simulink model "Test_model_nou"  (R2023b)
settings: Solver=ode15s  StartTime=0.0  StopTime=10  RelTol=1e-3
values from neighbouring files (symbols this model uses):
  Ts = 0.1    [NonLinearARXModel.mat]    (also in NonLinearHammerstein-Weiner.mat; Workspace.mat)
settings Model: Creator=petri  LastModifiedBy=petri

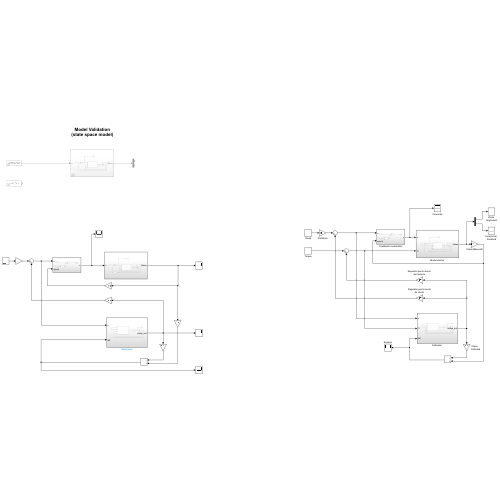
[thumbnail: Simulink's stored preview of the top-level diagram]
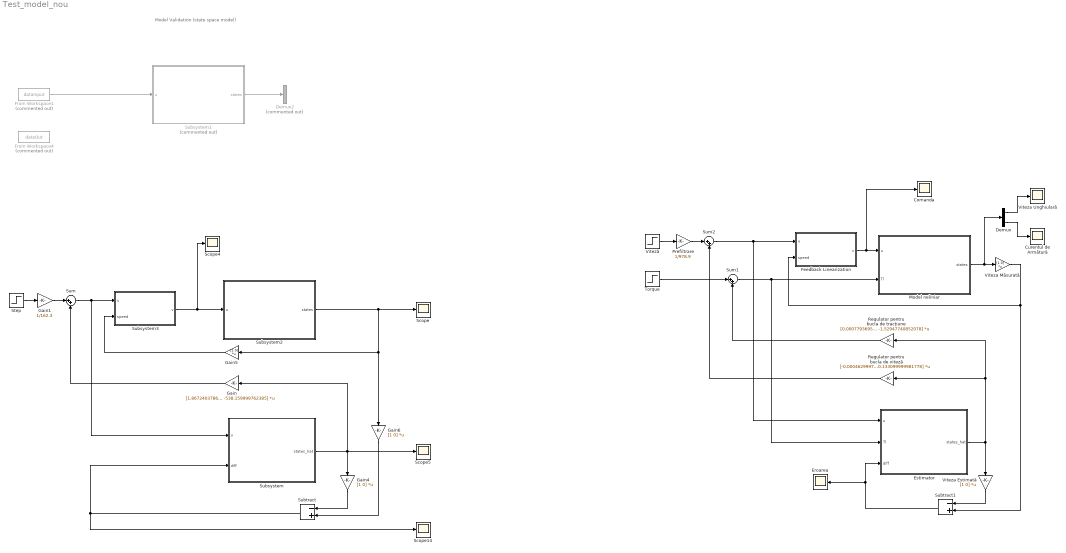
== system Test_model_nou ==
  note: Model Validation
      | (state space model)
  Comanda : Scope
  Curentul de Armătură : Scope
  Demux : Demux  Outputs=2
  Demux2 : Demux  Commented=on  Outputs=2
  Eroarea : Scope
  "Estimator " : Subsystem
  Feedback Linearization : Subsystem
  From Workspace1 : FromWorkspace  Commented=on  VariableName=dataInput  SampleTime=Ts
  From Workspace4 : FromWorkspace  Commented=on  VariableName=dataOut  SampleTime=Ts
  Gain : Gain  Gain=[1.86724037861208 -538.159999762385]  Multiplication=Matrix(K*u)
  Gain1 : Gain  Gain=1/162.3
  Gain4 : Gain  Gain=[1 0]  Multiplication=Matrix(K*u)
  Gain5 : Gain  Gain=[1 0]  Multiplication=Matrix(K*u)
  Gain6 : Gain  Gain=[1 0]  Multiplication=Matrix(K*u)
  Model neliniar : Subsystem
  Prefiltrare : Gain  Gain=1/978.9
  Regulator pentru bucla de viteză : Gain  Gain="[-0.000462999781953050\t0.133099999981778]"  Multiplication=Matrix(K*u)
  Regulator pentru bucla de tracțiune : Gain  Gain="[0.000779369551615828\t-1.52947740852078]"  Multiplication=Matrix(K*u)
  Scope{,4..5,14} (4 alike) : Scope
  Step : Step  Time=0  After=200  SampleTime=0
  Subsystem : Subsystem
  Subsystem1 : Subsystem  Commented=on
  Subsystem2 : Subsystem
  Subsystem3 : Subsystem
  Subtract : Sum  Inputs=-+
  Subtract1 : Sum  Inputs=-+
  Sum : Sum  Inputs=|++
  Sum1 : Sum  Inputs=|++
  Sum2 : Sum  Inputs=|++
  Torque : Step  Time=5  After=0.05  SampleTime=0
  Viteza Estimată : Gain  Gain=[1 0]  Multiplication=Matrix(K*u)
  Viteza Unghiulară : Scope
  Viteza Măsurată : Gain  Gain=[1 0]  Multiplication=Matrix(K*u)
  Viteză : Step  Time=0  After=160  SampleTime=0
  wires:
  From Workspace1/1 -> Subsystem1/1(u)
  Subsystem1/1(states) -> Demux2/1
  Subsystem3/1(v) -> Scope4/1, Subsystem2/1(u)
  Subsystem2/1(states) -> Scope/1, Gain6/1, Gain5/1
  Sum/1 -> Subsystem3/1(u), Subsystem/1(u)
  Gain/1 -> Sum/2
  Gain5/1 -> Subsystem3/2(speed)
  Subsystem/1(states_hat) -> Gain/1, Scope5/1, Gain4/1
  Gain4/1 -> Subtract/1
  Gain6/1 -> Subtract/2
  Subtract/1 -> Subsystem/2(diff), Scope14/1
  Step/1 -> Gain1/1
  Gain1/1 -> Sum/1
  Feedback Linearization/1(v) -> Model neliniar/1(u), Comanda/1
  Model neliniar/1(states) -> Viteza Măsurată/1, Demux/1
  Sum1/1 -> Model neliniar/2(Tl), "Estimator "/2(Tl)
  Sum2/1 -> "Estimator "/1(u), Feedback Linearization/1(u)
  Regulator pentru bucla de viteză/1 -> Sum2/2
  "Estimator "/1(states_hat) -> Viteza Estimată/1, Regulator pentru bucla de viteză/1, Regulator pentru bucla de tracțiune/1
  Viteza Estimată/1 -> Subtract1/1
  Viteza Măsurată/1 -> Feedback Linearization/2(speed), Subtract1/2
  Subtract1/1 -> Eroarea/1, "Estimator "/3(diff)
  Viteză/1 -> Prefiltrare/1
  Prefiltrare/1 -> Sum2/1
  Demux/1 -> Viteza Unghiulară/1
  Demux/2 -> Curentul de Armătură/1
  Regulator pentru bucla de tracțiune/1 -> Sum1/2
  Torque/1 -> Sum1/1

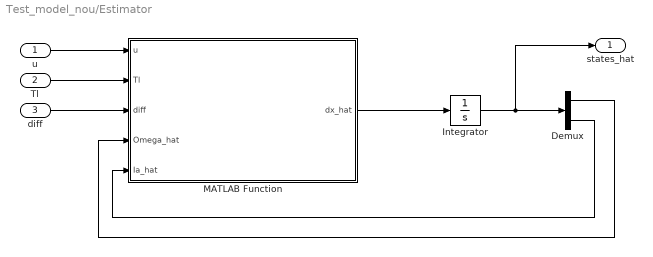
== system Test_model_nou/Estimator  ==
  u : Inport
  Tl : Inport  Port=2
  diff : Inport  Port=3
  Demux : Demux  Outputs=2
  Integrator : Integrator
  MATLAB Function : MATLAB Function  TreatAsAtomicUnit=on
  states_hat : Outport
  wires:
  u/1 -> MATLAB Function/1(u)
  Integrator/1 -> states_hat/1, Demux/1
  MATLAB Function/1(dx_hat) -> Integrator/1
  diff/1 -> MATLAB Function/3(diff)
  Demux/1 -> MATLAB Function/4(Omega_hat)
  Demux/2 -> MATLAB Function/5(Ia_hat)
  Tl/1 -> MATLAB Function/2(Tl)

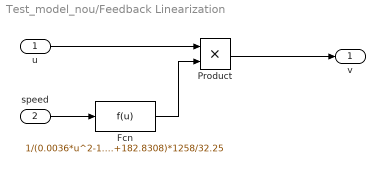
== system Test_model_nou/Feedback Linearization ==
  u : Inport
  speed : Inport  Port=2
  Fcn : Fcn  Expr=1/(0.0036*u^2-1.4479*u+182.8308)*1258/32.25
  Product : Product
  v : Outport
  wires:
  u/1 -> Product/1
  Fcn/1 -> Product/2
  speed/1 -> Fcn/1
  Product/1 -> v/1

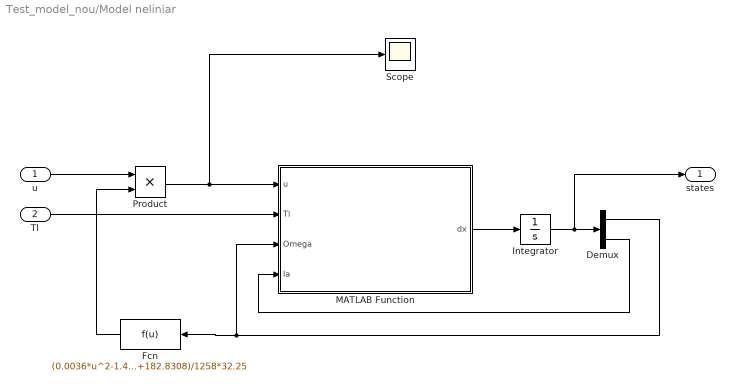
== system Test_model_nou/Model neliniar ==
  u : Inport
  Tl : Inport  Port=2
  Demux : Demux  Outputs=2
  Fcn : Fcn  Expr=(0.0036*u^2-1.4479*u+182.8308)/1258*32.25
  Integrator : Integrator
  MATLAB Function : MATLAB Function  TreatAsAtomicUnit=on
  Product : Product
  Scope : Scope
  states : Outport
  wires:
  Integrator/1 -> states/1, Demux/1
  Demux/2 -> MATLAB Function/4(Ia)
  MATLAB Function/1(dx) -> Integrator/1
  Demux/1 -> Fcn/1, MATLAB Function/3(Omega)
  u/1 -> Product/1
  Product/1 -> Scope/1, MATLAB Function/1(u)
  Fcn/1 -> Product/2
  Tl/1 -> MATLAB Function/2(Tl)

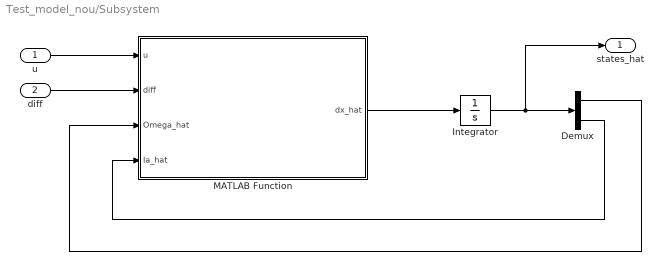
== system Test_model_nou/Subsystem ==
  u : Inport
  diff : Inport  Port=2
  Demux : Demux  Outputs=2
  Integrator : Integrator
  MATLAB Function : MATLAB Function  TreatAsAtomicUnit=on
  states_hat : Outport
  wires:
  u/1 -> MATLAB Function/1(u)
  Integrator/1 -> states_hat/1, Demux/1
  MATLAB Function/1(dx_hat) -> Integrator/1
  diff/1 -> MATLAB Function/2(diff)
  Demux/1 -> MATLAB Function/3(Omega_hat)
  Demux/2 -> MATLAB Function/4(Ia_hat)

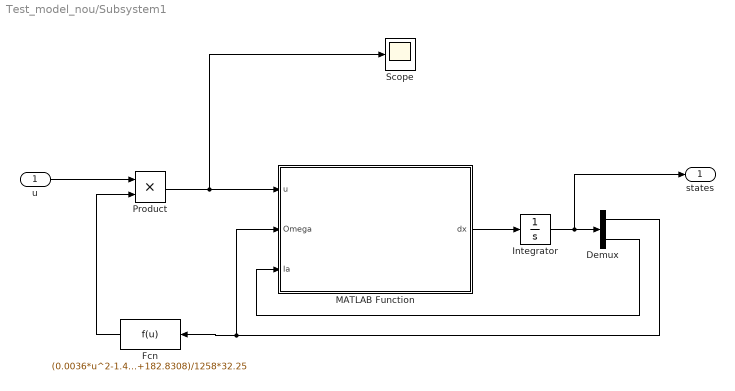
== system Test_model_nou/Subsystem1 ==
  u : Inport
  Demux : Demux  Outputs=2
  Fcn : Fcn  Expr=(0.0036*u^2-1.4479*u+182.8308)/1258*32.25
  Integrator : Integrator
  MATLAB Function : MATLAB Function  TreatAsAtomicUnit=on
  Product : Product
  Scope : Scope
  states : Outport
  wires:
  Integrator/1 -> states/1, Demux/1
  Demux/2 -> MATLAB Function/3(Ia)
  MATLAB Function/1(dx) -> Integrator/1
  Demux/1 -> Fcn/1, MATLAB Function/2(Omega)
  u/1 -> Product/1
  Product/1 -> MATLAB Function/1(u), Scope/1
  Fcn/1 -> Product/2

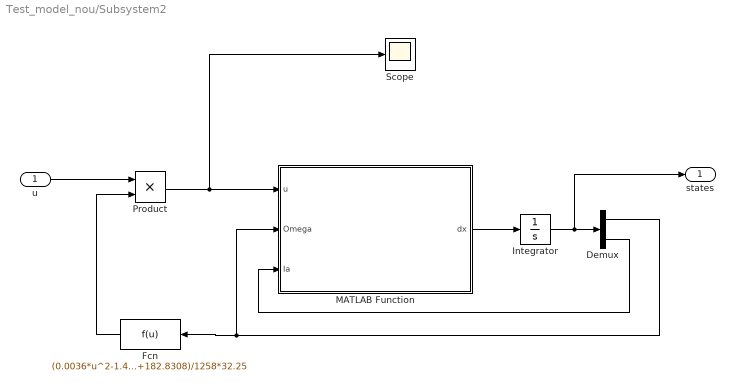
== system Test_model_nou/Subsystem2 ==
  u : Inport
  Demux : Demux  Outputs=2
  Fcn : Fcn  Expr=(0.0036*u^2-1.4479*u+182.8308)/1258*32.25
  Integrator : Integrator
  MATLAB Function : MATLAB Function  TreatAsAtomicUnit=on
  Product : Product
  Scope : Scope
  states : Outport
  wires:
  Integrator/1 -> states/1, Demux/1
  Demux/2 -> MATLAB Function/3(Ia)
  MATLAB Function/1(dx) -> Integrator/1
  Demux/1 -> Fcn/1, MATLAB Function/2(Omega)
  u/1 -> Product/1
  Product/1 -> Scope/1, MATLAB Function/1(u)
  Fcn/1 -> Product/2

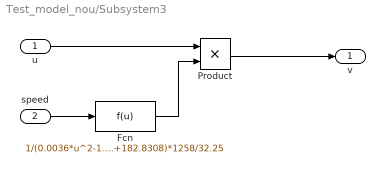
== system Test_model_nou/Subsystem3 ==
  u : Inport
  speed : Inport  Port=2
  Fcn : Fcn  Expr=1/(0.0036*u^2-1.4479*u+182.8308)*1258/32.25
  Product : Product
  v : Outport
  wires:
  u/1 -> Product/1
  Fcn/1 -> Product/2
  speed/1 -> Fcn/1
  Product/1 -> v/1

== matlab function Test_model_nou/Subsystem1/MATLAB Function ==
  data: u input; dx output; Omega input; Ia input
function dx = model(u, Omega, Ia)
J = 5.99e-8;
Ke = 0.0039;
Kf = 0.00291;
Kt = 0.1331;
Ra = 0.05;
La = 0.1;
x = [Omega; Ia];
A = [-Kf/J Kt/J*2*pi; -Ke/La/2/pi -Ra/La];
B = [0; 1/La];
dx = A*x+B*u;

== matlab function Test_model_nou/Subsystem2/MATLAB Function ==
  data: u input; dx output; Omega input; Ia input
function dx = model(u, Omega, Ia)
J = 5.99e-8;
Ke = 0.0039;
Kf = 0.00291;
Kt = 0.1331;
Ra = 0.05;
La = 0.1;
x = [Omega; Ia];
A = [-Kf/J Kt/J*2*pi; -Ke/La/2/pi -Ra/La];
B = [0; 1/La];
dx = A*x+B*u;

== matlab function Test_model_nou/Subsystem/MATLAB Function ==
  data: u input; dx_hat output; diff input; Omega_hat input; Ia_hat input
function dx_hat = estimator(u, diff, Omega_hat, Ia_hat)
A =[-48580.9682804674 13961468.5206278;-0.00620704278058392	-0.500000000000000];
B = [0; 10];
L = [48581.4682804675;0.0221007564488399];
x_hat = [Omega_hat; Ia_hat];
dx_hat = A*x_hat + B*u + L*diff;

== matlab function Test_model_nou/Model neliniar/MATLAB Function ==
  data: u input; Tl input; dx output; Omega input; Ia input
function dx = model(u, Tl, Omega, Ia)
J = 5.99e-8;
Ke = 0.0039;
Kf = 0.00291;
Kt = 0.1331;
Ra = 0.05;
La = 0.1;
U = [Tl; u];
x = [Omega; Ia];
A = [-Kf/J Kt/J*2*pi; -Ke/La/2/pi -Ra/La];
B = [-1/J*2*pi 0; 0 1/La];
dx = A*x+B*U;

== matlab function Test_model_nou/Estimator /MATLAB Function ==
  data: u input; Tl input; dx_hat output; diff input; Omega_hat input; Ia_hat input
function dx_hat = estimator(u, Tl, diff, Omega_hat, Ia_hat)
A = [-48580.9682804674 13961468.5206278;-0.00620704278058392	-0.500000000000000];
B = [-104894579.418691 0; 0 10];
L = [437233.214524207; 0.771081144725617];
%L = [48581.4682804675;0.0221007564488399];
U = [Tl;u];
x_hat = [Omega_hat; Ia_hat];
dx_hat = A*x_hat + B*U + L*diff;
